simulink model "Inverted_pendulum_angle_ctrlCopyInCaseSomethingGoesWrong"  (R2023a)
settings: Solver=ode45  StartTime=0  StopTime=T_f  MaxStep=MaxStep  RelTol=RelTol  AbsTol=1e-6
undefined symbols (not defined in the file): A_alpha, A_ctrl, b, B_alpha_1, B_alpha_2, B_ctrl, C_ctrl, D_ctrl, g, Ja, Jb, k, l, M, ma, mb, omega0, T_f, theta0, v0, x0
Description:
  | Inverted Pendulum with Animation
  | 
  | This example shows how to model an inverted pendulum.  The animation is created using MATLAB(R) Handle Graphics(R).  The animation block is a masked
  | S-function.  For more information, use the context menu to look under the Animation block's mask
  | and open the S-function for editing.
settings Model: Creator=The MathWorks, Inc.  LastModifiedBy=matte
settings SolverCC: AutoScaleAbsTol=off  AlgebraicLoopSolver=TrustRegion
settings DataIOCC: ExternalInput=[]  InitialState=[]  SaveFormat=Array  SaveOutput=off  SaveTime=off  ReturnWorkspaceOutputs=off
settings OptimizationCC: BlockReduction=off  BooleanDataType=off  ReuseModelBlockBuffer=off  ExpressionDepthLimit=2147483647  InitFltsAndDblsToZero=on  LifeSpan=inf
settings DebuggingCC: SaveWithParameterizedLinksMsg=none  UnderspecifiedInitializationDetection=Classic  MergeDetectMultiDrivingBlocksExec=none  SignalResolutionControl=TryResolveAllWithWarning  MultiTaskDSMMsg=warning  MultiTaskCondExecSysMsg=none  SigSpecEnsureSampleTimeMsg=none  FcnCallInpInsideContextMsg=warning  UnconnectedInputMsg=warning  UnconnectedOutputMsg=warning  UnconnectedLineMsg=warning  StateNameClashWarn=warning  SFUnexpectedBacktrackingDiag=warning  SFNoUnconditionalDefaultTransitionDiag=warning  SFExecutionAtInitializationDiag=none  ArithmeticOperatorsInVariantConditions=warning
settings HardwareCC: ProdBitPerPointer=32  ProdBitPerSizeT=32  ProdBitPerPtrDiffT=32  ProdLargestAtomicFloat=None  ProdIntDivRoundTo=Undefined  ProdEndianess=Unspecified  ProdWordSize=32  ProdHWDeviceType=32-bit Generic  TargetUnknown=on
settings ModelReferenceCC: EnableRefExpFcnMdlSchedulingChecks=on  PropagateSignalLabelsOutOfModel=off
settings SFSimCC: SimUseLocalCustomCode=off  CustomCodeUndefinedFunction=UseInterfaceOnly
settings RTWCC: RTWUseLocalCustomCode=off
settings CodeAppCC: StateflowObjectComments=on
settings GRTTargetCC: TargetFcnLib=ansi_tfl_tmw.mat  TargetLangStandard=C89/C90 (ANSI)  CombineOutputUpdateFcns=off  GRTInterface=on
settings ConfigComp: CovMetricSettings=dw  CovSaveCumulativeToWorkspaceVar=on  CovSaveSingleToWorkspaceVar=on  CovExternalEMLEnable=off

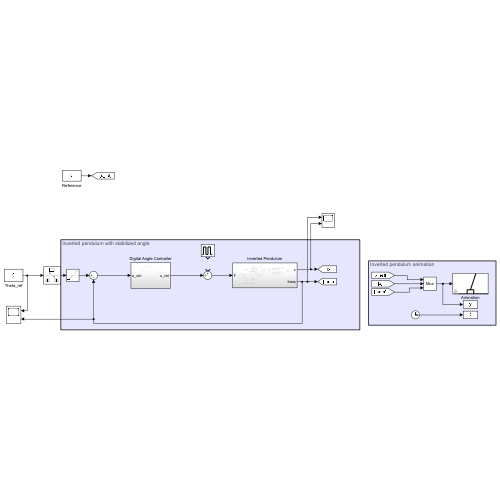
[thumbnail: Simulink's stored preview of the top-level diagram]
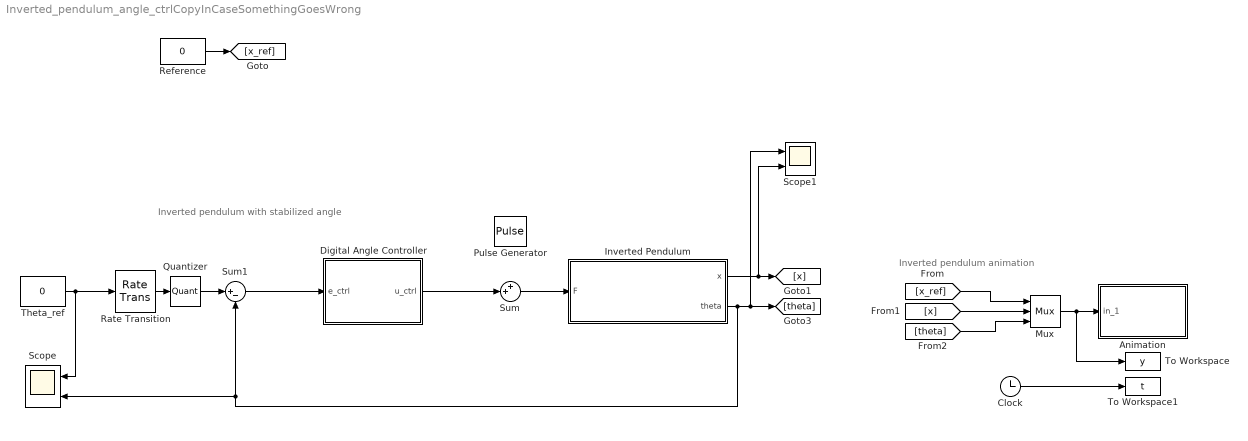
== system Inverted_pendulum_angle_ctrlCopyInCaseSomethingGoesWrong ==
  note: Inverted pendulum with stabilized angle
  note: Inverted pendulum animation
  Animation : Subsystem  mask(Pendulum plot){RefBlock=Reference}
      mask prompts: RefBlock "DC reference signal block name:"
      mask help: Pendulum plot
      mask Help: Pendulum animation function using Handle graphics.
      mask Display: plot([-10 10],[0 0],[-2 -2 2 2],[0 1 1 0],[0 3],[1 5])
  Clock : Clock
  Digital Angle Controller : Subsystem
  Inverted Pendulum : Subsystem
  Mux : Mux  Inputs=3
  Pulse Generator : DiscretePulseGenerator  PulseType=Time based  Amplitude=1000  Period=10  PulseWidth=0.01
  Quantizer : Quantizer  QuantizationInterval=2*pi/(2^T_f)
  Rate Transition : RateTransition  Integrity=off  OutPortSampleTime=Ts
  Reference : Constant  Value=0
  Scope : Scope  NumInputPorts=2
  Scope1 : Scope  NumInputPorts=2
  Sum : Sum  Inputs=++|
  Sum1 : Sum  Inputs=|+-
  Theta_ref : Constant  Value=0
  To Workspace : ToWorkspace  VariableName=y  SampleTime=0.02
  To Workspace1 : ToWorkspace  VariableName=t  SampleTime=0.02
  wires:
  Reference/1 -> [x_ref]
  [x_ref] -> Mux/1
  [x] -> Mux/2
  [theta] -> Mux/3
  Mux/1 -> To Workspace/1, Animation/1(in_1)
  Clock/1 -> To Workspace1/1
  Inverted Pendulum/1(x) -> Scope1/2, [x]
  Digital Angle Controller/1(u_ctrl) -> Sum/2
  Sum/1 -> Inverted Pendulum/1(F)
  Sum1/1 -> Digital Angle Controller/1(e_ctrl)
  Inverted Pendulum/2(theta) -> Sum1/2, Scope/2, Scope1/1, [theta]
  Theta_ref/1 -> Scope/1, Rate Transition/1
  Rate Transition/1 -> Quantizer/1
  Quantizer/1 -> Sum1/1

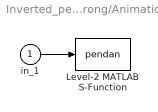
== system Inverted_pendulum_angle_ctrlCopyInCaseSomethingGoesWrong/Animation ==
  in_1 : Inport
  Level-2 MATLAB S-Function : M-S-Function  FunctionName=pendan  Parameters=RefBlock
  wires:
  in_1/1 -> Level-2 MATLAB S-Function/1

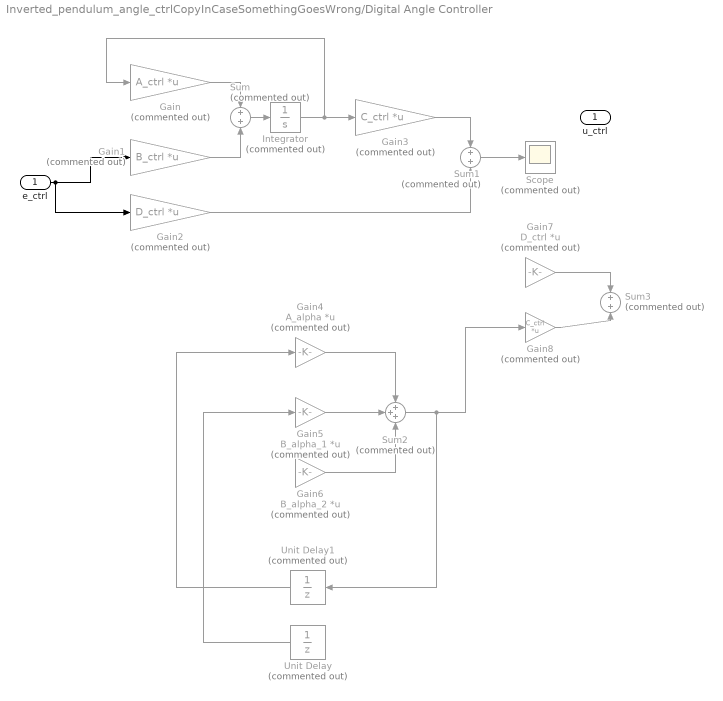
== system Inverted_pendulum_angle_ctrlCopyInCaseSomethingGoesWrong/Digital Angle Controller ==
  e_ctrl : Inport
  Gain : Gain  Commented=on  Gain=A_ctrl  Multiplication=Matrix(K*u)
  Gain1 : Gain  Commented=on  Gain=B_ctrl  Multiplication=Matrix(K*u)
  Gain2 : Gain  Commented=on  Gain=D_ctrl  Multiplication=Matrix(K*u)
  Gain3 : Gain  Commented=on  Gain=C_ctrl  Multiplication=Matrix(K*u)
  Gain4 : Gain  Commented=on  Gain=A_alpha  Multiplication=Matrix(K*u)
  Gain5 : Gain  Commented=on  Gain=B_alpha_1  Multiplication=Matrix(K*u)
  Gain6 : Gain  Commented=on  Gain=B_alpha_2  Multiplication=Matrix(K*u)
  Gain7 : Gain  Commented=on  Gain=D_ctrl  Multiplication=Matrix(K*u)
  Gain8 : Gain  Commented=on  Gain=C_ctrl  Multiplication=Matrix(K*u)
  Integrator : Integrator  Commented=on
  Scope : Scope  Commented=on
  Sum : Sum  Commented=on
  Sum1 : Sum  Commented=on
  Sum2 : Sum  Commented=on  Inputs=+++
  Sum3 : Sum  Commented=on  Inputs=+|+
  Unit Delay : UnitDelay  Commented=on  SampleTime=-1  HasFrameUpgradeWarning=on
  Unit Delay1 : UnitDelay  Commented=on  SampleTime=-1  HasFrameUpgradeWarning=on
  u_ctrl : Outport
  wires:
  Sum/1 -> Integrator/1
  Gain/1 -> Sum/1
  Integrator/1 -> Gain3/1, Gain/1
  Gain1/1 -> Sum/2
  Sum1/1 -> Scope/1
  Gain3/1 -> Sum1/1
  Gain2/1 -> Sum1/2
  Gain5/1 -> Sum2/2
  Gain4/1 -> Sum2/1
  Gain6/1 -> Sum2/3
  Sum2/1 -> Unit Delay1/1, Gain8/1
  Unit Delay1/1 -> Gain4/1
  Unit Delay/1 -> Gain5/1
  Gain7/1 -> Sum3/1
  Gain8/1 -> Sum3/2
  e_ctrl/1 -> Gain2/1, Gain1/1

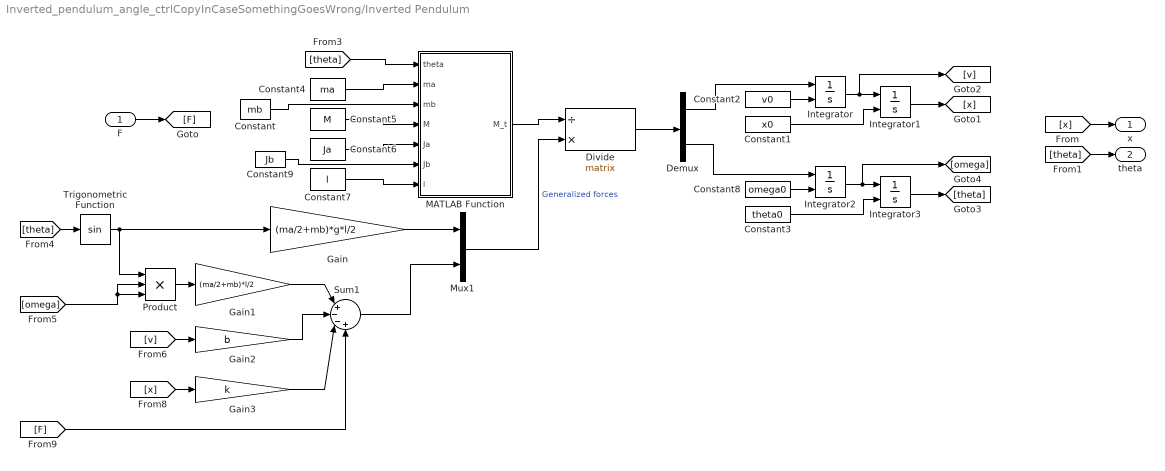
== system Inverted_pendulum_angle_ctrlCopyInCaseSomethingGoesWrong/Inverted Pendulum ==
  F : Inport
  Constant : Constant  Value=mb
  Constant1 : Constant  Value=x0
  Constant2 : Constant  Value=v0
  Constant3 : Constant  Value=theta0
  Constant4 : Constant  Value=ma
  Constant5 : Constant  Value=M
  Constant6 : Constant  Value=Ja
  Constant7 : Constant  Value=l
  Constant8 : Constant  Value=omega0
  Constant9 : Constant  Value=Jb
  Demux : Demux  Outputs=2
  Divide : Product  Inputs=/*  Multiplication=Matrix(*)
  Gain : Gain  Gain=(ma/2+mb)*g*l/2
  Gain1 : Gain  Gain=(ma/2+mb)*l/2
  Gain2 : Gain  Gain=b
  Gain3 : Gain  Gain=k
  Integrator : Integrator  InitialConditionSource=external
  Integrator1 : Integrator  InitialConditionSource=external
  Integrator2 : Integrator  InitialConditionSource=external
  Integrator3 : Integrator  InitialConditionSource=external  WrapState=on
  MATLAB Function : MATLAB Function  TreatAsAtomicUnit=on
  Mux1 : Mux  Inputs=2
  Product : Product  Inputs=3
  Sum1 : Sum  Inputs=|+--+
  Trigonometric Function : Trigonometry
  x : Outport
  theta : Outport  Port=2
  wires:
  Integrator/1 -> [v], Integrator1/1
  Integrator3/1 -> [theta]
  [omega] -> Product/2, Product/3
  Integrator1/1 -> [x]
  Integrator2/1 -> [omega], Integrator3/1
  Divide/1 -> Demux/1
  Demux/2 -> Integrator2/1
  Gain2/1 -> Sum1/2
  Sum1/1 -> Mux1/2
  [theta] -> Trigonometric Function/1
  Product/1 -> Gain1/1
  MATLAB Function/1(M_t) -> Divide/1
  Gain/1 -> Mux1/1
  Trigonometric Function/1 -> Gain/1, Product/1
  Mux1/1 -> Divide/2  "Generalized forces"
  [F] -> Sum1/4
  Gain1/1 -> Sum1/1
  Constant2/1 -> Integrator/2
  Constant3/1 -> Integrator3/2
  [x] -> Gain3/1
  Demux/1 -> Integrator/1
  Gain3/1 -> Sum1/3
  [v] -> Gain2/1
  Constant1/1 -> Integrator1/2
  F/1 -> [F]
  [x] -> x/1
  [theta] -> theta/1
  Constant8/1 -> Integrator2/2
  [theta] -> MATLAB Function/1(theta)
  Constant4/1 -> MATLAB Function/2(ma)
  Constant5/1 -> MATLAB Function/4(M)
  Constant/1 -> MATLAB Function/3(mb)
  Constant6/1 -> MATLAB Function/5(Ja)
  Constant9/1 -> MATLAB Function/6(Jb)
  Constant7/1 -> MATLAB Function/7(l)

== matlab function Inverted_pendulum_angle_ctrlCopyInCaseSomethingGoesWrong/Inverted Pendulum/MATLAB Function ==
  data: theta input; M_t output; ma input; mb input; M input; Ja input; Jb input; l input
function M_t = Inertia(theta, ma, mb, M, Ja, Jb, l)
%% Computation of the inertia matrix
M_t = [(ma/2+mb)*l*cos(theta) (ma/4+mb)*l^2+Ja+Jb;
            M+ma+mb (ma/2+mb)*l*cos(theta)];
